simulink model "UNIFIER_ROMdyn"  (R2023b)
settings: Solver=VariableStepAuto  StartTime=0.0  StopTime=0  RelTol=1e-3
libraries: aerolibatmos2 x1
settings Model: Creator=Reggie Johanes  LastModifiedBy=Reggie Johanes

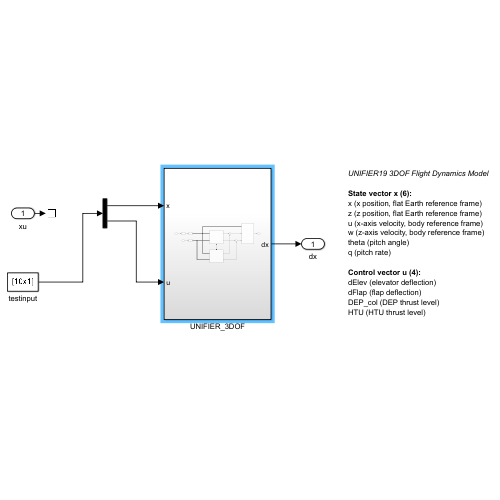
[thumbnail: Simulink's stored preview of the top-level diagram]
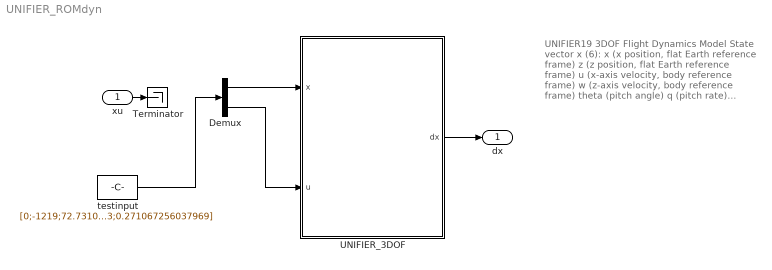
== system UNIFIER_ROMdyn ==
  note: UNIFIER19 3DOF Flight Dynamics Model
      |
      | State vector x (6):
      | x (x position, flat Earth reference frame)
      | z (z position, flat Earth reference frame)
      | u (x-axis velocity, body reference frame)
      | w (z-axis velocity, body reference frame)
      | theta (pitch angle)
      | q (pitch rate)
      |
      | Control vector u (4):
      | dElev (elevator deflection)
      | dFlap (flap deflection)
      | DEP_col (DEP thrust level)
      | HTU (HTU thrust level)
  xu : Inport
  Demux : Demux  Outputs=[6,4]
  Terminator : Terminator
  UNIFIER_3DOF : Subsystem
  testinput : Constant  Value=[0;-1219;72.731047032614440;1.142307104518741;0.015706052282666;0;-0.015298320692100;0;0.306978739246813;0.271067256037969]
  dx : Outport
  wires:
  UNIFIER_3DOF/1(dx) -> dx/1
  xu/1 -> Terminator/1
  testinput/1 -> Demux/1
  Demux/1 -> UNIFIER_3DOF/1(x)
  Demux/2 -> UNIFIER_3DOF/2(u)

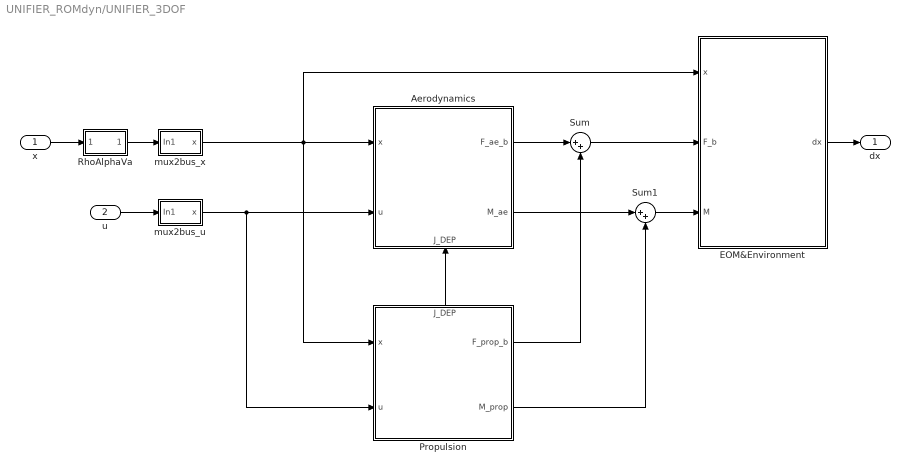
== system UNIFIER_ROMdyn/UNIFIER_3DOF ==
  x : Inport
  u : Inport  Port=2
  Aerodynamics : Subsystem
      settings: PortSchema="{\"entries\":[{\"content\":{\"sides\":[{\"content\":{\"connectorIds\":[\"In1\",\"In2\"]},\"type\":\"ConnectorPlacement.EquallySpacedRectSide\",\"uuid\":\"17ee4459-7bca-4fc7-ac8a-5f8d484d0f96\"},{\"content\":{\"connectorIds\":[\"Out1\",\"Out2\"],\"side\":\"RIGHT\"},\"type\":\"ConnectorPlacement.EquallySpacedRectSide\",\"uuid\":\"9b92559e-06f7-4af4-8484-f34dac8672b4\"},{\"content\":{\"side\":\"TOP\"},\"type\":\"ConnectorPlacement.EquallySpacedRectSide\",\"uuid\":\"a4f2e9fa-eae6-474f-ad2c-489301d84b22\"},{\"content\":{\"connectorIds\":[\"In3\"],\"side\":\"BOTTOM\"},\"type\":\"ConnectorPlacement.EquallySpacedRectSide\",\"uuid\":\"178ea2f1-e4a2-458b-b79e-a56beb6169b5\"}]},\"type\":\"ConnectorPlacement.EquallySpacedConnector\",\"uuid\":\"479c014a-6cba-4ef7-bfe0-51bf14fc9f63\"}],\"packageUris\":[\"http://schema.mathworks.com/mf0/Connector/R2020b\"],\"version\":\"1.0\"}"
  EOM&Environment : Subsystem
  Propulsion : Subsystem
      settings: PortSchema="{\"entries\":[{\"content\":{\"sides\":[{\"content\":{\"connectorIds\":[\"In1\",\"In2\"]},\"type\":\"ConnectorPlacement.EquallySpacedRectSide\",\"uuid\":\"07d6f334-da9b-43bc-8919-35c75dc56ebf\"},{\"content\":{\"connectorIds\":[\"Out1\",\"Out2\"],\"side\":\"RIGHT\"},\"type\":\"ConnectorPlacement.EquallySpacedRectSide\",\"uuid\":\"71e67728-3303-46b8-a0cb-58b7e4eaf9eb\"},{\"content\":{\"connectorIds\":[\"Out3\"],\"side\":\"TOP\"},\"type\":\"ConnectorPlacement.EquallySpacedRectSide\",\"uuid\":\"b3b60b63-634a-4790-bc05-b0be525e2f04\"}]},\"type\":\"ConnectorPlacement.EquallySpacedConnector\",\"uuid\":\"5a9d657d-d483-47e8-9c23-43355ba90f0d\"}],\"packageUris\":[\"http://schema.mathworks.com/mf0/Connector/R2020b\"],\"version\":\"1.0\"}"
  RhoAlphaVa : Subsystem
  Sum : Sum  Inputs=|++
  Sum1 : Sum  Inputs=|++
  mux2bus_u : Subsystem
  mux2bus_x : Subsystem
  dx : Outport
  wires:
  u/1 -> mux2bus_u/1(In1)
  x/1 -> RhoAlphaVa/1(In1)
  Aerodynamics/1(F_ae_b) -> Sum/1
  Sum/1 -> EOM&Environment/2(F_b)
  Propulsion/1(F_prop_b) -> Sum/2
  Aerodynamics/2(M_ae) -> Sum1/1
  Sum1/1 -> EOM&Environment/3(M)
  Propulsion/2(M_prop) -> Sum1/2
  EOM&Environment/1(dx) -> dx/1
  RhoAlphaVa/1(Out1) -> mux2bus_x/1(In1)
  mux2bus_x/1(x) -> EOM&Environment/1(x), Aerodynamics/1(x), Propulsion/1(x)
  mux2bus_u/1(x) -> Aerodynamics/2(u), Propulsion/2(u)
  Propulsion/3(J_DEP) -> Aerodynamics/3(J_DEP)

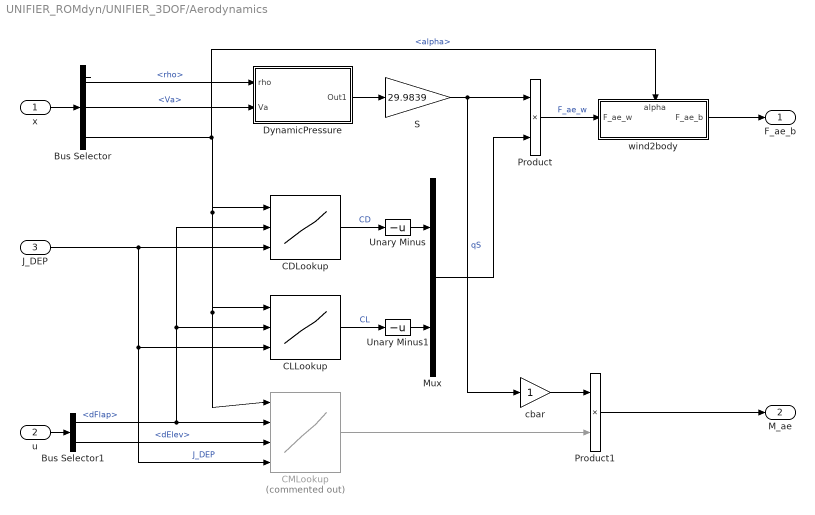
== system UNIFIER_ROMdyn/UNIFIER_3DOF/Aerodynamics ==
  x : Inport
  u : Inport  Port=2
  J_DEP : Inport  Port=3
  Bus Selector : BusSelector  OutputSignals=rho,Va,alpha
  Bus Selector1 : BusSelector  OutputSignals=dFlap,dElev
  CDLookup : Lookup_n-D  NumberOfTableDimensions=3  BreakpointsForDimension3=[5, 7]  Table=reshape(repmat([4 5 6;16 19 20;10 18 23],1,2),[3,3,2])  InternalRulePriority=Speed  RndMeth=Simplest
      settings: InputPortMap=u0,u1,u2
  CLLookup : Lookup_n-D  NumberOfTableDimensions=3  BreakpointsForDimension3=[5, 7]  Table=reshape(repmat([4 5 6;16 19 20;10 18 23],1,2),[3,3,2])  InternalRulePriority=Speed  RndMeth=Simplest
      settings: InputPortMap=u0,u1,u2
  CMLookup : Lookup_n-D  Commented=on  NumberOfTableDimensions=4  BreakpointsForDimension3=[5, 7]  Table=reshape(repmat([4 5 6;16 19 20;10 18 23],1,2),[3,3,2])  InternalRulePriority=Speed  RndMeth=Simplest
      settings: InputPortMap=u0,u1,u2,u3
  DynamicPressure : Subsystem
  Mux : Mux  Inputs=2
  Product : Product
  Product1 : Product
  S : Gain  Gain=29.9839
  Unary Minus : UnaryMinus
  Unary Minus1 : UnaryMinus
  cbar : Gain
  wind2body : Subsystem
      settings: PortSchema="{\"entries\":[{\"content\":{\"sides\":[{\"content\":{\"connectorIds\":[\"In1\"]},\"type\":\"ConnectorPlacement.EquallySpacedRectSide\",\"uuid\":\"290c73ed-3dea-48ea-8152-da6c73d4cb7e\"},{\"content\":{\"connectorIds\":[\"Out1\"],\"side\":\"RIGHT\"},\"type\":\"ConnectorPlacement.EquallySpacedRectSide\",\"uuid\":\"998f7612-46b2-4329-a1d2-339c41b842ac\"},{\"content\":{\"connectorIds\":[\"In2\"],\"side\":\"TOP\"},\"type\":\"ConnectorPlacement.EquallySpacedRectSide\",\"uuid\":\"f5aa2474-eb99-4d6b-9b61-1c1ef88f9e9d\"}]},\"type\":\"ConnectorPlacement.EquallySpacedConnector\",\"uuid\":\"e9cadda8-b54c-4a15-b91d-81264397230a\"}],\"packageUris\":[\"http://schema.mathworks.com/mf0/Connector/R2020b\"],\"version\":\"1.0\"}"
  F_ae_b : Outport
  M_ae : Outport  Port=2
  wires:
  x/1 -> Bus Selector/1
  DynamicPressure/1(Out1) -> S/1
  u/1 -> Bus Selector1/1
  Bus Selector1/1 -> CDLookup/2, CLLookup/2, CMLookup/2  "<dFlap>"
  Bus Selector/2 -> DynamicPressure/2(Va)  "<Va>"
  Bus Selector/1 -> DynamicPressure/1(rho)  "<rho>"
  Bus Selector/3 -> wind2body/2(alpha), CDLookup/1, CMLookup/1, CLLookup/1  "<alpha>"
  S/1 -> Product/1, cbar/1  "qS"
  Bus Selector1/2 -> CMLookup/3  "<dElev>"
  J_DEP/1 -> CDLookup/3, CMLookup/4, CLLookup/3  "J_DEP"
  CDLookup/1 -> Unary Minus/1  "CD"
  Product/1 -> wind2body/1(F_ae_w)  "F_ae_w"
  CLLookup/1 -> Unary Minus1/1  "CL"
  Unary Minus/1 -> Mux/1
  Unary Minus1/1 -> Mux/2
  Mux/1 -> Product/2
  wind2body/1(F_ae_b) -> F_ae_b/1
  CMLookup/1 -> Product1/2
  cbar/1 -> Product1/1
  Product1/1 -> M_ae/1

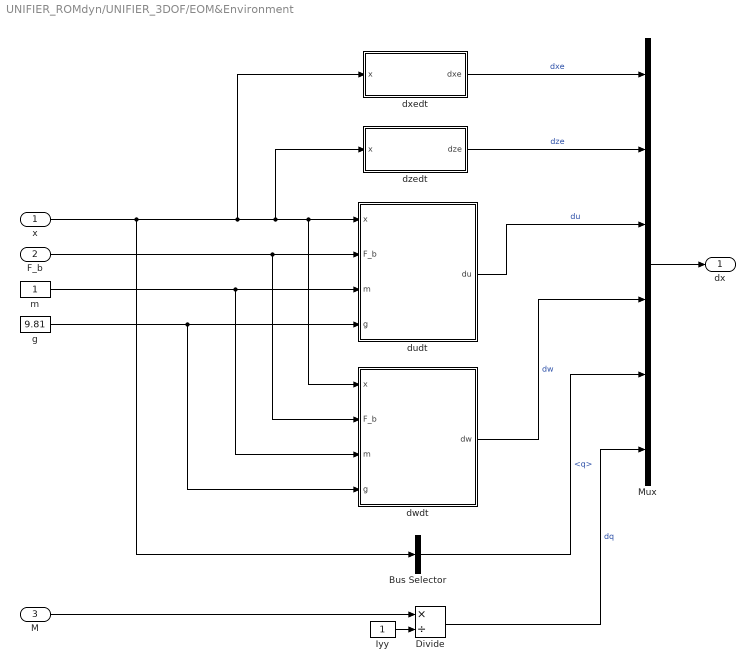
== system UNIFIER_ROMdyn/UNIFIER_3DOF/EOM&Environment ==
  x : Inport
  F_b : Inport  Port=2
  M : Inport  Port=3
  Bus Selector : BusSelector  OutputSignals=q
  Divide : Product  Inputs=*/
  Iyy : Constant
  Mux : Mux  Inputs=6
  dudt : Subsystem
  dwdt : Subsystem
  dxedt : Subsystem
  dzedt : Subsystem
  g : Constant  Value=9.81
  m : Constant
  dx : Outport
  wires:
  M/1 -> Divide/1
  Iyy/1 -> Divide/2
  Mux/1 -> dx/1
  Divide/1 -> Mux/6  "dq"
  x/1 -> Bus Selector/1, dxedt/1(x), dzedt/1(x), dwdt/1(x), dudt/1(x)
  F_b/1 -> dwdt/2(F_b), dudt/2(F_b)
  m/1 -> dwdt/3(m), dudt/3(m)
  g/1 -> dwdt/4(g), dudt/4(g)
  dudt/1(du) -> Mux/3  "du"
  dxedt/1(dxe) -> Mux/1  "dxe"
  dzedt/1(dze) -> Mux/2  "dze"
  dwdt/1(dw) -> Mux/4  "dw"
  Bus Selector/1 -> Mux/5  "<q>"

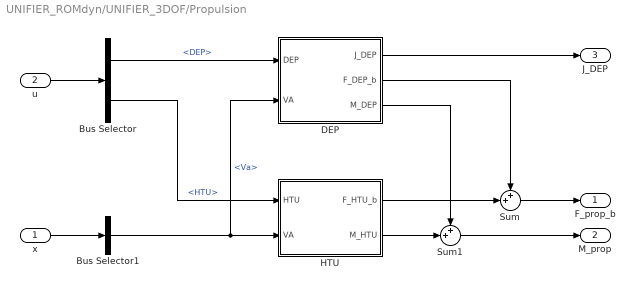
== system UNIFIER_ROMdyn/UNIFIER_3DOF/Propulsion ==
  x : Inport
  u : Inport  Port=2
  Bus Selector : BusSelector  OutputSignals=DEP,HTU
  Bus Selector1 : BusSelector  OutputSignals=Va
  DEP : Subsystem
  HTU : Subsystem
  Sum : Sum  Inputs=++|
  Sum1 : Sum  Inputs=++|
  F_prop_b : Outport
  M_prop : Outport  Port=2
  J_DEP : Outport  Port=3
  wires:
  u/1 -> Bus Selector/1
  x/1 -> Bus Selector1/1
  Bus Selector1/1 -> DEP/2(VA), HTU/2(VA)  "<Va>"
  Bus Selector/1 -> DEP/1(DEP)  "<DEP>"
  Bus Selector/2 -> HTU/1(HTU)  "<HTU>"
  DEP/1(J_DEP) -> J_DEP/1
  HTU/2(M_HTU) -> Sum1/2
  HTU/1(F_HTU_b) -> Sum/2
  DEP/2(F_DEP_b) -> Sum/1
  DEP/3(M_DEP) -> Sum1/1
  Sum/1 -> F_prop_b/1
  Sum1/1 -> M_prop/1

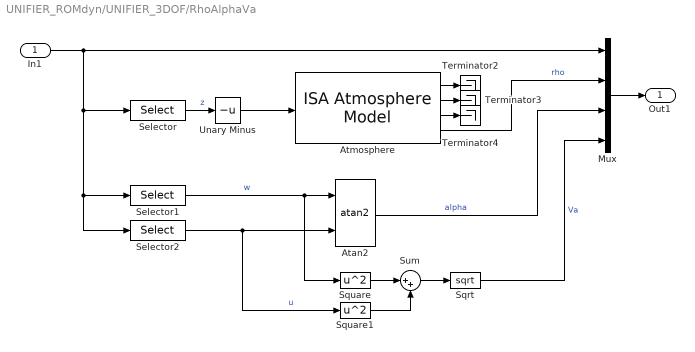
== system UNIFIER_ROMdyn/UNIFIER_3DOF/RhoAlphaVa ==
  In1 : Inport
  Atan2 : Trigonometry  Operator=atan2
  Atmosphere : aerolibatmos2/ISA Atmosphere Model  useExtended=off  action=Warning  custom=off  viscosityOut=off  g=9.80665  gamma=1.4  R=287.0531  L=0.0065  h_trop=11000  h_strat=20000  rho0=1.225  P0=101325  T0=288.15  h0=0
  Mux : Mux
  Selector : Selector  InputPortWidth=6  IndexOptions=Index vector (dialog)  Indices=2  OutputSizes=1
  Selector1 : Selector  InputPortWidth=6  IndexOptions=Index vector (dialog)  Indices=4  OutputSizes=1
  Selector2 : Selector  InputPortWidth=6  IndexOptions=Index vector (dialog)  Indices=3  OutputSizes=1
  Sqrt : Sqrt
  Square : Math  Operator=square
  Square1 : Math  Operator=square
  Sum : Sum  Inputs=|++
  Terminator2 : Terminator
  Terminator3 : Terminator
  Terminator4 : Terminator
  Unary Minus : UnaryMinus
  Out1 : Outport
  wires:
  In1/1 -> Selector2/1, Selector1/1, Selector/1, Mux/1
  Selector/1 -> Unary Minus/1  "z"
  Unary Minus/1 -> Atmosphere/1
  Atmosphere/3 -> Terminator4/1
  Atmosphere/4 -> Mux/2  "rho"
  Atmosphere/2 -> Terminator3/1
  Atmosphere/1 -> Terminator2/1
  Mux/1 -> Out1/1
  Selector2/1 -> Square1/1, Atan2/2  "u"
  Atan2/1 -> Mux/3  "alpha"
  Sum/1 -> Sqrt/1
  Square1/1 -> Sum/2
  Selector1/1 -> Square/1, Atan2/1  "w"
  Square/1 -> Sum/1
  Sqrt/1 -> Mux/4  "Va"

== system UNIFIER_ROMdyn/UNIFIER_3DOF/mux2bus_u ==
  In1 : Inport
  Bus Creator : BusCreator  Inputs=4
  Demux : Demux
  x : Outport
  wires:
  In1/1 -> Demux/1
  Demux/2 -> Bus Creator/2  "dFlap"
  Demux/3 -> Bus Creator/3  "DEP"
  Demux/1 -> Bus Creator/1  "dElev"
  Bus Creator/1 -> x/1
  Demux/4 -> Bus Creator/4  "HTU"

== system UNIFIER_ROMdyn/UNIFIER_3DOF/mux2bus_x ==
  In1 : Inport
  Bus Creator : BusCreator  Inputs=9
  Demux : Demux  Outputs=9
  x : Outport
  wires:
  In1/1 -> Demux/1
  Bus Creator/1 -> x/1
  Demux/1 -> Bus Creator/1  "xe"
  Demux/2 -> Bus Creator/2  "ze"
  Demux/3 -> Bus Creator/3  "u"
  Demux/4 -> Bus Creator/4  "w"
  Demux/5 -> Bus Creator/5  "theta"
  Demux/6 -> Bus Creator/6  "q"
  Demux/7 -> Bus Creator/7  "rho"
  Demux/8 -> Bus Creator/8  "alpha"
  Demux/9 -> Bus Creator/9  "Va"

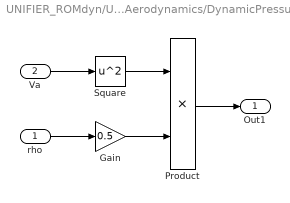
== system UNIFIER_ROMdyn/UNIFIER_3DOF/Aerodynamics/DynamicPressure ==
  rho : Inport
  Va : Inport  Port=2
  Gain : Gain  Gain=0.5
  Product : Product
  Square : Math  Operator=square
  Out1 : Outport
  wires:
  Va/1 -> Square/1
  rho/1 -> Gain/1
  Square/1 -> Product/1
  Gain/1 -> Product/2
  Product/1 -> Out1/1

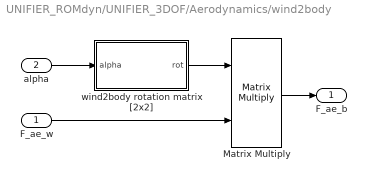
== system UNIFIER_ROMdyn/UNIFIER_3DOF/Aerodynamics/wind2body ==
  F_ae_w : Inport
  alpha : Inport  Port=2
  Matrix Multiply : Product  Multiplication=Matrix(*)
  wind2body rotation matrix [2x2] : MATLAB Function  TreatAsAtomicUnit=on
  F_ae_b : Outport
  wires:
  alpha/1 -> wind2body rotation matrix [2x2]/1(alpha)
  wind2body rotation matrix [2x2]/1(rot) -> Matrix Multiply/1
  F_ae_w/1 -> Matrix Multiply/2
  Matrix Multiply/1 -> F_ae_b/1

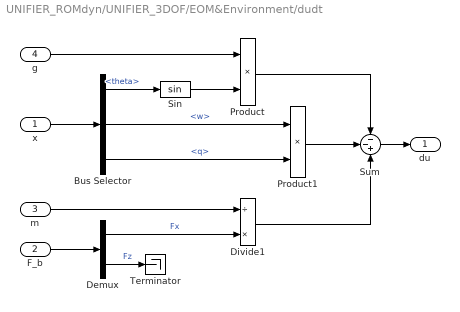
== system UNIFIER_ROMdyn/UNIFIER_3DOF/EOM&Environment/dudt ==
  x : Inport
  F_b : Inport  Port=2
  m : Inport  Port=3
  g : Inport  Port=4
  Bus Selector : BusSelector  OutputSignals=theta,w,q
  Demux : Demux  Outputs=2
  Divide1 : Product  Inputs=/*
  Product : Product
  Product1 : Product
  Sin : Trigonometry
  Sum : Sum  Inputs=--+
  Terminator : Terminator
  du : Outport
  wires:
  Product/1 -> Sum/1
  Sin/1 -> Product/2
  Bus Selector/2 -> Product1/1  "<w>"
  Bus Selector/1 -> Sin/1  "<theta>"
  Bus Selector/3 -> Product1/2  "<q>"
  Product1/1 -> Sum/2
  Demux/2 -> Terminator/1  "Fz"
  x/1 -> Bus Selector/1
  F_b/1 -> Demux/1
  g/1 -> Product/1
  m/1 -> Divide1/1
  Sum/1 -> du/1
  Demux/1 -> Divide1/2  "Fx"
  Divide1/1 -> Sum/3

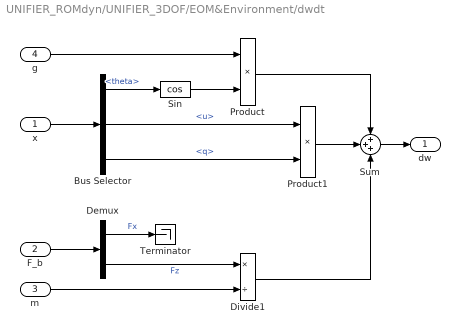
== system UNIFIER_ROMdyn/UNIFIER_3DOF/EOM&Environment/dwdt ==
  x : Inport
  F_b : Inport  Port=2
  m : Inport  Port=3
  g : Inport  Port=4
  Bus Selector : BusSelector  OutputSignals=theta,u,q
  Demux : Demux  Outputs=2
  Divide1 : Product  Inputs=*/
  Product : Product
  Product1 : Product
  Sin : Trigonometry  Operator=cos
  Sum : Sum  Inputs=+++
  Terminator : Terminator
  dw : Outport
  wires:
  Product/1 -> Sum/1
  Sin/1 -> Product/2
  Bus Selector/2 -> Product1/1  "<u>"
  Bus Selector/1 -> Sin/1  "<theta>"
  Bus Selector/3 -> Product1/2  "<q>"
  Product1/1 -> Sum/2
  Demux/2 -> Divide1/1  "Fz"
  x/1 -> Bus Selector/1
  F_b/1 -> Demux/1
  g/1 -> Product/1
  m/1 -> Divide1/2
  Sum/1 -> dw/1
  Demux/1 -> Terminator/1  "Fx"
  Divide1/1 -> Sum/3

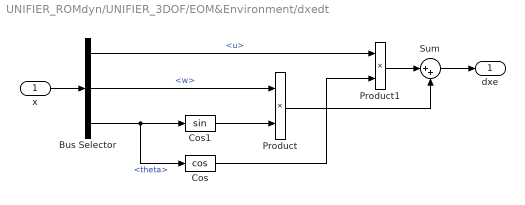
== system UNIFIER_ROMdyn/UNIFIER_3DOF/EOM&Environment/dxedt ==
  x : Inport
  Bus Selector : BusSelector  OutputSignals=u,w,theta
  Cos : Trigonometry  Operator=cos
  Cos1 : Trigonometry
  Product : Product
  Product1 : Product
  Sum : Sum  Inputs=|++
  dxe : Outport
  wires:
  x/1 -> Bus Selector/1
  Bus Selector/1 -> Product1/1  "<u>"
  Bus Selector/2 -> Product/1  "<w>"
  Bus Selector/3 -> Cos/1, Cos1/1  "<theta>"
  Cos1/1 -> Product/2
  Cos/1 -> Product1/2
  Product/1 -> Sum/2
  Product1/1 -> Sum/1
  Sum/1 -> dxe/1

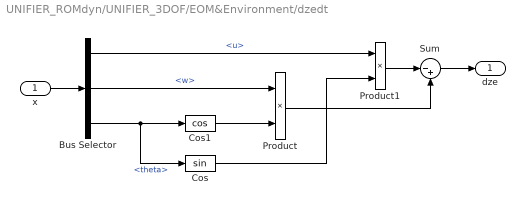
== system UNIFIER_ROMdyn/UNIFIER_3DOF/EOM&Environment/dzedt ==
  x : Inport
  Bus Selector : BusSelector  OutputSignals=u,w,theta
  Cos : Trigonometry
  Cos1 : Trigonometry  Operator=cos
  Product : Product
  Product1 : Product
  Sum : Sum  Inputs=|-+
  dze : Outport
  wires:
  x/1 -> Bus Selector/1
  Bus Selector/1 -> Product1/1  "<u>"
  Bus Selector/2 -> Product/1  "<w>"
  Bus Selector/3 -> Cos/1, Cos1/1  "<theta>"
  Cos1/1 -> Product/2
  Cos/1 -> Product1/2
  Product/1 -> Sum/2
  Product1/1 -> Sum/1
  Sum/1 -> dze/1

== system UNIFIER_ROMdyn/UNIFIER_3DOF/Propulsion/DEP ==
  DEP : Inport
  VA : Inport  Port=2
  J_DEP : Outport
  F_DEP_b : Outport  Port=2
  M_DEP : Outport  Port=3

== system UNIFIER_ROMdyn/UNIFIER_3DOF/Propulsion/HTU ==
  HTU : Inport
  VA : Inport  Port=2
  F_HTU_b : Outport
  M_HTU : Outport  Port=2

== matlab function UNIFIER_ROMdyn/UNIFIER_3DOF/Aerodynamics/wind2body/wind2body rotation matrix [2x2] ==
  data: alpha input; rot output
function rot = fcn(alpha)

rot = [cos(alpha) -sin(alpha);
       sin(alpha)  cos(alpha)];

end
